simulink model "robotReferenceTrackingMarch"  (R2020a)
settings: Solver=ode1  StartTime=0.0  StopTime=10.0  FixedStep=0.001  MaxStep=0.01  RelTol=1e-3  EnableMultiTasking=on
values from neighbouring files (symbols this model uses):
  a11 = -70/3085    (= -0.0226904376013)    [tracking_1.m]
  ac = -1    [tracking_1.m]
  b1 = 1/3085    (= 0.00032414910859)    [tracking_1.m]
  F = [K 1]*inv(TT)    [tracking_2.m]
  G = Gr*inv(TT1(:,nn-pp+1:nn))    [tracking_2.m]
  Y_v_bar = -992/3085    (= -0.321555915721)    [tracking_1.m]
settings Model: Creator=xiaoran  LastModifiedBy=xiaoran
settings DataIOCC: LimitDataPoints=on  SaveFormat=Array  ReturnWorkspaceOutputs=off
settings OptimizationCC: LifeSpan=inf
settings DebuggingCC: UnderspecifiedInitializationDetection=Classic  MergeDetectMultiDrivingBlocksExec=none  SolverPrmCheckMsg=warning  StateNameClashWarn=warning  SFUnexpectedBacktrackingDiag=warning  SFNoUnconditionalDefaultTransitionDiag=warning  SFExecutionAtInitializationDiag=none  ArithmeticOperatorsInVariantConditions=warning
settings HardwareCC: ProdBitPerPointer=32  ProdBitPerSizeT=32  ProdBitPerPtrDiffT=32  ProdLargestAtomicFloat=None  ProdIntDivRoundTo=Undefined  ProdEndianess=Unspecified  ProdWordSize=32  ProdHWDeviceType=32-bit Generic
settings ModelReferenceCC: PropagateSignalLabelsOutOfModel=off
settings SFSimCC: SimUseLocalCustomCode=off  CustomCodeUndefinedFunction=UseInterfaceOnly
settings RTWCC: RTWUseLocalCustomCode=off
settings CodeAppCC: StateflowObjectComments=on
settings GRTTargetCC: TargetLangStandard=C89/C90 (ANSI)
settings ConfigComp: CovMetricSettings=dw  CovHtmlReporting=on  CovSaveCumulativeToWorkspaceVar=on  CovSaveSingleToWorkspaceVar=on  CovExternalEMLEnable=off

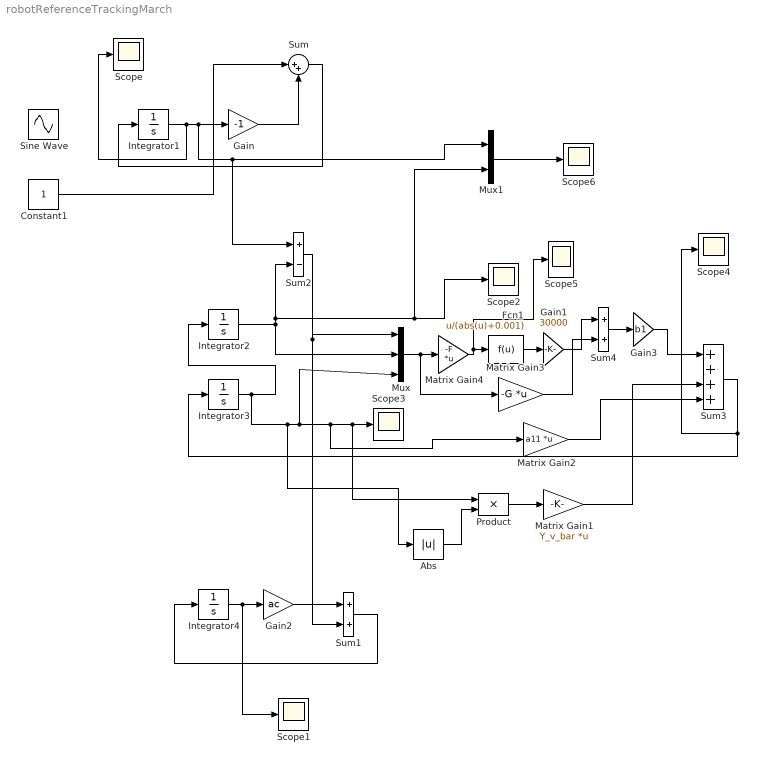
== system robotReferenceTrackingMarch ==
  Abs : Abs
  Constant1 : Constant
  Fcn1 : Fcn  Expr=u/(abs(u)+0.001)
  Gain : Gain  Gain=-1
  Gain1 : Gain  Gain=30000  SaturateOnIntegerOverflow=on  OutDataTypeStr=Inherit: Same as input  ParamDataTypeStr=Inherit: Same as input
  Gain2 : Gain  Gain=ac
  Gain3 : Gain  Gain=b1  SaturateOnIntegerOverflow=on  OutDataTypeStr=Inherit: Same as input  ParamDataTypeStr=Inherit: Same as input
  Integrator1 : Integrator  InitialCondition=0.1
  Integrator2 : Integrator  InitialCondition=0.1
  Integrator3 : Integrator
  Integrator4 : Integrator  InitialCondition=0.1
  Matrix Gain1 : Gain  Gain=Y_v_bar  Multiplication=Matrix(K*u)  SaturateOnIntegerOverflow=on  OutDataTypeStr=Inherit: Same as input  ParamDataTypeStr=Inherit: Same as input
  Matrix Gain2 : Gain  Gain=a11  Multiplication=Matrix(K*u)  SaturateOnIntegerOverflow=on  OutDataTypeStr=Inherit: Same as input  ParamDataTypeStr=Inherit: Same as input
  Matrix Gain3 : Gain  Gain=-G  Multiplication=Matrix(K*u)  SaturateOnIntegerOverflow=on  OutDataTypeStr=Inherit: Same as input  ParamDataTypeStr=Inherit: Same as input
  Matrix Gain4 : Gain  Gain=-F  Multiplication=Matrix(K*u)  SaturateOnIntegerOverflow=on  OutDataTypeStr=Inherit: Same as input  ParamDataTypeStr=Inherit: Same as input
  Mux : Mux  Inputs=3
  Mux1 : Mux  Inputs=2
  Product : Product
  Scope{,1..6} (7 alike) : Scope
  Sine Wave : Sin  SampleTime=0
  Sum : Sum  Inputs=|++
  Sum1 : Sum  InputSameDT=on  SaturateOnIntegerOverflow=on  OutDataTypeStr=Inherit: Same as first input
  Sum2 : Sum  Inputs=+-  InputSameDT=on  SaturateOnIntegerOverflow=on  OutDataTypeStr=Inherit: Same as first input
  Sum3 : Sum  Inputs=++++  InputSameDT=on  SaturateOnIntegerOverflow=on  OutDataTypeStr=Inherit: Same as first input
  Sum4 : Sum  InputSameDT=on  SaturateOnIntegerOverflow=on  OutDataTypeStr=Inherit: Same as first input
  wires:
  Integrator1/1 -> Scope/1, Mux1/1, Sum2/1, Gain/1
  Gain/1 -> Sum/2
  Sum/1 -> Integrator1/1
  Integrator2/1 -> Scope2/1, Mux1/2, Sum2/2, Mux/2
  Integrator3/1 -> Abs/1, Mux/3, Matrix Gain2/1, Product/1, Scope3/1, Integrator2/1
  Fcn1/1 -> Gain1/1
  Matrix Gain4/1 -> Fcn1/1, Scope5/1
  Mux/1 -> Matrix Gain3/1, Matrix Gain4/1
  Sum3/1 -> Scope4/1, Integrator3/1
  Mux1/1 -> Scope6/1
  Sum2/1 -> Mux/1, Sum1/2
  Constant1/1 -> Sum/1
  Integrator4/1 -> Scope1/1, Gain2/1
  Gain2/1 -> Sum1/1
  Sum1/1 -> Integrator4/1
  Abs/1 -> Product/2
  Product/1 -> Matrix Gain1/1
  Matrix Gain1/1 -> Sum3/3
  Matrix Gain2/1 -> Sum3/4
  Gain1/1 -> Sum4/1
  Matrix Gain3/1 -> Sum4/2
  Sum4/1 -> Gain3/1
  Gain3/1 -> Sum3/1
